simulink model "phase1_PRControl_CIM_noAdapt"  (R2024a)
settings: Solver=VariableStepAuto  StartTime=0.0  StopTime=3  FixedStep=1e-7  MaxStep=1e-6  RelTol=1e-6
values from neighbouring files (symbols this model uses):
  Cf = 22e-6    (= 2.2e-05)    [phase1_PRControl_CIM_noAdapt_init.m]
  L1 = 150e-6    (= 0.00015)    [phase1_PRControl_CIM_noAdapt_init.m]
  L2g = L2+Lg    (= 0.00045)    [phase1_PRControl_CIM_noAdapt_init.m]
  R1 = 0.045    [phase1_PRControl_CIM_noAdapt_init.m]
  R2g = R2+Rg    (= 0.135)    [phase1_PRControl_CIM_noAdapt_init.m]
  Rd = 1    [phase1_PRControl_CIM_noAdapt_init.m]
  w = 2*pi*freq    (= 314.159265359)    [phase1_PRControl_CIM_noAdapt_init.m]
  w2 = 3*w    (= 942.477796077)    [phase1_PRControl_CIM_noAdapt_init.m]
libraries: spsVoltageMeasurementLib x4, spsSeriesRLCBranchLib x3, spsDCVoltageSourceLib x2, cstblocks x2, spsControlledVoltageSourceLib x1, spsCurrentMeasurementLib x1, spsBreakerLib x1, spsPLLLib x1, simulink x1, spsdq0toAlphaBetaZeroLib x1, spsUniversalBridgeLib x1, spspowerguiLib x1
settings Model: Creator=aleks  LastModifiedBy=aleks
settings DataIOCC: ReturnWorkspaceOutputs=off
settings SimscapeCC: SimscapeLogType=all  SimscapeLogOpenViewer=on  SimscapeLogLimitData=off

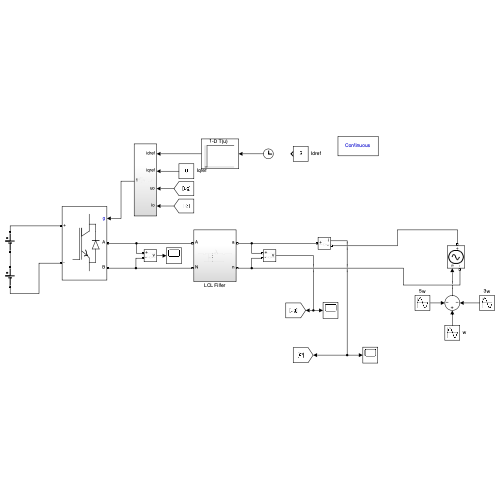
[thumbnail: Simulink's stored preview of the top-level diagram]
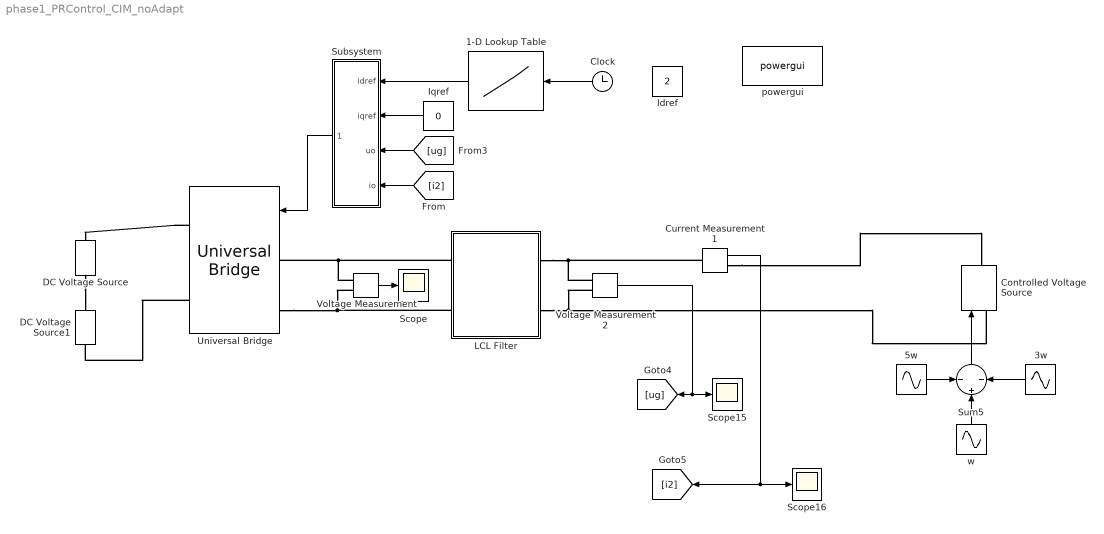
== system phase1_PRControl_CIM_noAdapt ==
  1-D Lookup Table : Lookup_n-D  NumberOfTableDimensions=1  LookupTableObject=''  BreakpointsForDimension1=[0;0.2;0.201;3]  BreakpointsForDimension1FirstPoint=10  BreakpointsForDimension2FirstPoint=10  BreakpointsForDimension1Spacing=12  BreakpointsForDimension2Spacing=12  IndexSearchMethod=Linear search  Table=[0;0;2;2]  DiagnosticForOutOfRangeInput=Error  InternalRulePriority=Speed  RndMeth=Simplest
  3w : Sin  Amplitude=1.5  Frequency=w2  SampleTime=0
  5w : Sin  Amplitude=1.5  Frequency=5*w  SampleTime=0
  Clock : Clock
  Controlled Voltage Source : spsControlledVoltageSourceLib/Controlled Voltage Source  Initialize=on  Source_Type=AC  Amplitude=0  Phase=0  Frequency=0  Measurements=None
  Current Measurement1 : spsCurrentMeasurementLib/Current Measurement  PhasorSimulation=off  OutputType=Complex  PSBequivalent=0
  DC Voltage Source : spsDCVoltageSourceLib/DC Voltage Source  Amplitude=20  Measurements=None
  DC Voltage Source1 : spsDCVoltageSourceLib/DC Voltage Source  Amplitude=20  Measurements=None
  Idref : Constant  Value=2
  Iqref : Constant  Value=0
  LCL Filter : Subsystem
  Scope : Scope
  Scope15 : Scope
  Scope16 : Scope
  Subsystem : Subsystem
  Sum5 : Sum  Inputs=-|+|-
  Universal Bridge : spsUniversalBridgeLib/Universal Bridge  Arms=2  SnubberResistance=1e5  SnubberCapacitance=inf  Device=IGBT / Diodes  Ron=1e-3  Lon=0  ForwardVoltages="[  0  0  ]"  ForwardVoltage=0  GTOparameters=[ 10e-6 , 20e-6 ]  IGBTparameters=[ 1e-6 , 2e-6 ]  Measurements=None  Measurements_2=None  converterType=Rectifier
  Voltage Measurement : spsVoltageMeasurementLib/Voltage Measurement  PhasorSimulation=off  OutputType=Complex  PSBequivalent=0
  Voltage Measurement2 : spsVoltageMeasurementLib/Voltage Measurement  PhasorSimulation=off  OutputType=Complex  PSBequivalent=0
  powergui : spspowerguiLib/powergui  Priority=1  SimulationMode=Continuous  SampleTime=10e-6  frequency=60  Iterations=50  frequencyindice=0  Pbase=100e6  ErrMax=1e-4  UnitsV=kV  UnitsW=MW  buscounter=0  FunctionMessages=off  echomessages=off  EnableUseOfTLC=off  CurrentSourceSwitches=off  DisableSnubberDevices=off  DisableRonSwitches=off  DisableVfSwitches=off  DisplayEquations=off  AutomaticDiscreteSolvers=off  SolverType=Tustin/Backward Euler (TBE)  Interpol=off  ExternalGateDelay=off  methode=off  Ts=100  x0status=blocks  SPID=on  SwTol=0  HookPort=off  NonlinearTolerance=1e-4  nMaxIteration=100  ContinueOnMaxIteration=off  RestoreLinks=warning  ResistiveCurrentMeasurement=off  Frange=[0:2:500]  Ylog=off  Xlog=on  ShowGrid=off  save=off  variable=ZData  structure=0  ZoomFFT=off  StartTime=0.0  cycles=1  DisplayStyle=1  fundamental=60  FreqAxis=off  MaxFrequency=1000  frequencyindicesteady=1  RmsSteady=1  display=off
  w : Sin  Amplitude=15  Frequency=w  SampleTime=0
  wires:
  Voltage Measurement/1 -> Scope/1
  Subsystem/1(1) -> Universal Bridge/1
  [i2] -> Subsystem/4(io)
  [ug] -> Subsystem/3(uo)
  Voltage Measurement2/1 -> [ug], Scope15/1
  Current Measurement1/1 -> Scope16/1, [i2]
  w/1 -> Sum5/2
  3w/1 -> Sum5/3
  5w/1 -> Sum5/1
  Sum5/1 -> Controlled Voltage Source/1
  Iqref/1 -> Subsystem/2(iqref)
  1-D Lookup Table/1 -> Subsystem/1(idref)
  Clock/1 -> 1-D Lookup Table/1
  connections:
  Universal Bridge/RConn1 -- DC Voltage Source/RConn1
  Universal Bridge/RConn2 -- DC Voltage Source1/LConn1
  Voltage Measurement/LConn1 -- LCL Filter/LConn1 -- Universal Bridge/LConn1
  Voltage Measurement2/LConn2 -- Controlled Voltage Source/LConn1 -- LCL Filter/RConn2
  DC Voltage Source/LConn1 -- DC Voltage Source1/RConn1
  Voltage Measurement2/LConn1 -- LCL Filter/RConn1 -- Current Measurement1/LConn1
  Voltage Measurement/LConn2 -- LCL Filter/LConn2 -- Universal Bridge/LConn2
  Current Measurement1/RConn1 -- Controlled Voltage Source/RConn1

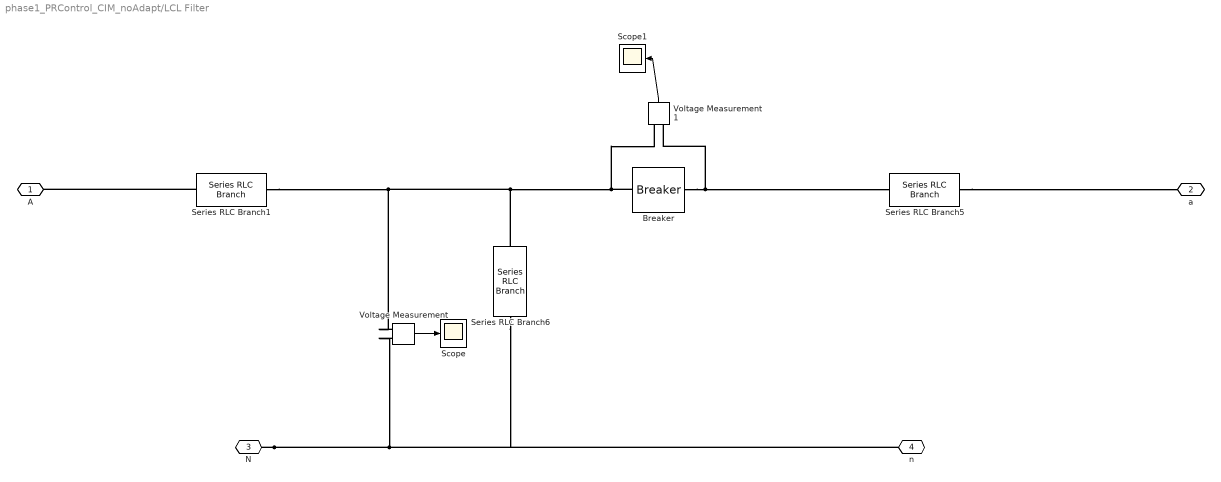
== system phase1_PRControl_CIM_noAdapt/LCL Filter ==
  Breaker : spsBreakerLib/Breaker  InitialState=0  SwitchingTimes=[0.1]  External=off  BreakerResistance=0.0001  SnubberResistance=1e8  SnubberCapacitance=inf  Measurements=None  MoreParameters=on  NoBreakLoop=off
  Scope : Scope
  Scope1 : Scope
  Series RLC Branch1 : spsSeriesRLCBranchLib/Series RLC Branch  LConnTagsString=__new0  RConnTagsString=__new0  BranchType=RL  Resistance=R1  Inductance=L1  SetiL0=off  InitialCurrent=0  Capacitance=1e-6  Setx0=off  InitialVoltage=0  Measurements=None
  Series RLC Branch5 : spsSeriesRLCBranchLib/Series RLC Branch  LConnTagsString=__new0  RConnTagsString=__new0  BranchType=RL  Resistance=R2g  Inductance=L2g  SetiL0=off  InitialCurrent=0  Capacitance=1e-6  Setx0=off  InitialVoltage=0  Measurements=None
  Series RLC Branch6 : spsSeriesRLCBranchLib/Series RLC Branch  LConnTagsString=__new0  RConnTagsString=__new0  BranchType=RC  Resistance=Rd  Inductance=500e-6  SetiL0=off  InitialCurrent=0  Capacitance=Cf  Setx0=off  InitialVoltage=0  Measurements=None
  Voltage Measurement : spsVoltageMeasurementLib/Voltage Measurement  PhasorSimulation=off  OutputType=Complex  PSBequivalent=0
  Voltage Measurement1 : spsVoltageMeasurementLib/Voltage Measurement  PhasorSimulation=off  OutputType=Complex  PSBequivalent=0
  A : PMIOPort  Side=Left
  a : PMIOPort  Port=2  Side=Right
  N : PMIOPort  Port=3  Side=Left
  n : PMIOPort  Port=4  Side=Right
  wires:
  Voltage Measurement1/1 -> Scope1/1
  Voltage Measurement/1 -> Scope/1
  connections:
  N/RConn1 -- Series RLC Branch6/LConn1 -- n/RConn1 -- Voltage Measurement/LConn2
  Series RLC Branch5/RConn1 -- a/RConn1
  Series RLC Branch1/LConn1 -- A/RConn1
  Series RLC Branch6/RConn1 -- Voltage Measurement1/LConn2 -- Breaker/LConn1 -- Voltage Measurement/LConn1 -- Series RLC Branch1/RConn1
  Breaker/RConn1 -- Series RLC Branch5/LConn1 -- Voltage Measurement1/LConn1

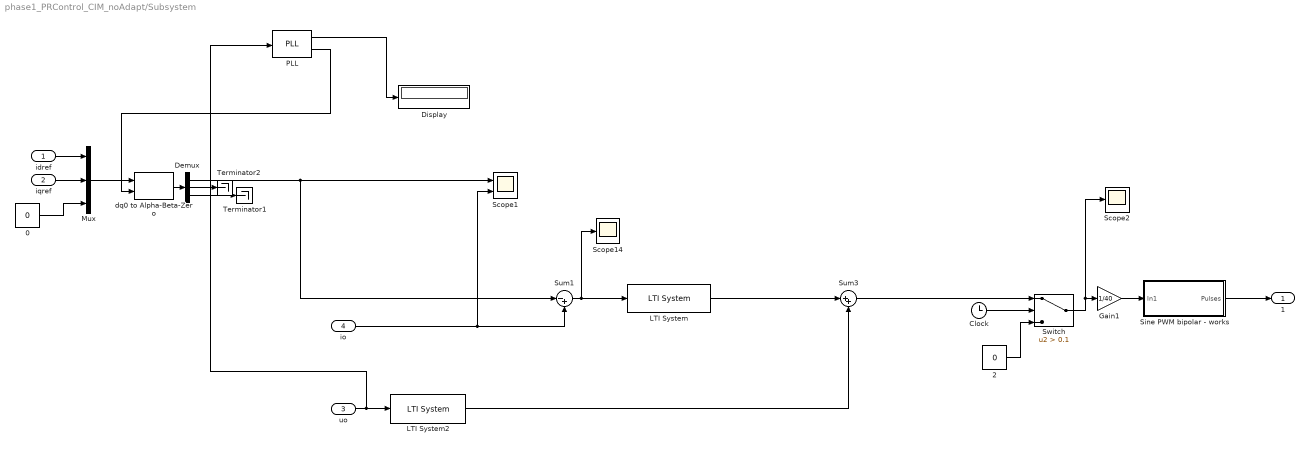
== system phase1_PRControl_CIM_noAdapt/Subsystem ==
  idref : Inport
  iqref : Inport  Port=2
  uo : Inport  Port=3
  io : Inport  Port=4
  0 : Constant  Value=0
  2 : Constant  Value=0
  Clock : Clock
  Demux : Demux  Outputs=3
  Display : Display
  Gain1 : Gain  Gain=1/40
  LTI System : cstblocks/LTI System  sys=R  IC=[]  PadeOrder=0
  LTI System2 : cstblocks/LTI System  sys=Gfffilter  IC=[]  PadeOrder=0
  Mux : Mux  Inputs=3
  PLL : spsPLLLib/PLL  Fmin=49  Par_Init=[0, 50]  ParK=[180, 3200, 1]  TcD=1e-4  MaxRateChangeFreq=12  FilterCutOffFreq=25  Ts=0  AGC=on
      settings: LibrarySourceBlock=sps_lib/Control/PLL
  Scope1 : Scope  NumInputPorts=2
  Scope14 : Scope
  Scope2 : Scope
  Sine PWM bipolar - works : Subsystem
  Sum1 : Sum  Inputs=|-+
  Sum3 : Sum  Inputs=|++
  Switch : Switch  Criteria=u2 > Threshold  Threshold=0.1  SaturateOnIntegerOverflow=off  InputSameDT=off
  Terminator1 : Terminator
  Terminator2 : Terminator
  dq0 to Alpha-Beta-Zero : spsdq0toAlphaBetaZeroLib/dq0 to Alpha-Beta-Zero  Alignment=90 degrees behind phase A axis
  1 : Outport
  wires:
  Demux/1 -> Sum1/1, Scope1/1
  io/1 -> Scope1/2, Sum1/2
  Sine PWM bipolar - works/1(Pulses) -> 1/1
  Gain1/1 -> Sine PWM bipolar - works/1(In1)
  Sum1/1 -> LTI System/1, Scope14/1
  LTI System2/1 -> Sum3/2
  LTI System/1 -> Sum3/1
  uo/1 -> PLL/1, LTI System2/1
  Mux/1 -> dq0 to Alpha-Beta-Zero/1
  0/1 -> Mux/3
  Demux/3 -> Terminator1/1
  Demux/2 -> Terminator2/1
  PLL/1 -> Display/1
  dq0 to Alpha-Beta-Zero/1 -> Demux/1
  PLL/2 -> dq0 to Alpha-Beta-Zero/2
  idref/1 -> Mux/1
  iqref/1 -> Mux/2
  2/1 -> Switch/3
  Clock/1 -> Switch/2
  Switch/1 -> Scope2/1, Gain1/1
  Sum3/1 -> Switch/1

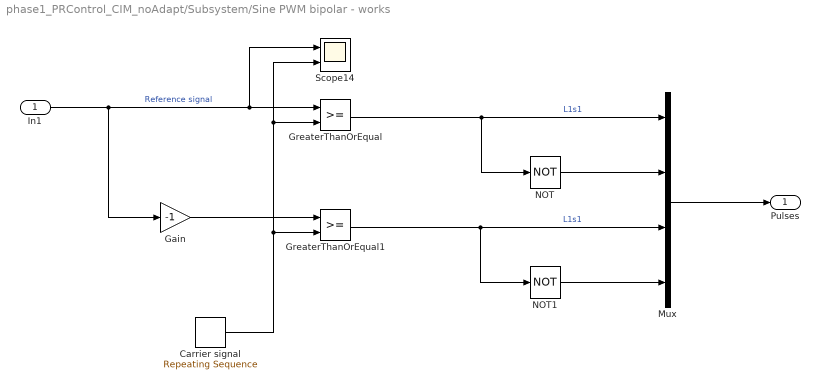
== system phase1_PRControl_CIM_noAdapt/Subsystem/Sine PWM bipolar - works ==
  In1 : Inport
  Carrier signal : simulink/Sources/Repeating Sequence  rep_seq_t=[0 1/24000 1/12000]  rep_seq_y=[-1 1 -1]
  Gain : Gain  Gain=-1
  GreaterThanOrEqual : RelationalOperator  OutDataTypeStr=boolean  RndMeth=Simplest  InputSameDT=off
  GreaterThanOrEqual1 : RelationalOperator  OutDataTypeStr=boolean  RndMeth=Simplest  InputSameDT=off
  Mux : Mux
  NOT : Logic  Operator=NOT  IconShape=distinctive  AllPortsSameDT=off  OutDataTypeStr=boolean
  NOT1 : Logic  Operator=NOT  IconShape=distinctive  AllPortsSameDT=off  OutDataTypeStr=boolean
  Scope14 : Scope  NumInputPorts=2
  Pulses : Outport
  wires:
  Mux/1 -> Pulses/1
  In1/1 -> Scope14/1, GreaterThanOrEqual/1, Gain/1  "Reference signal"
  Carrier signal/1 -> Scope14/2, GreaterThanOrEqual/2, GreaterThanOrEqual1/2
  GreaterThanOrEqual/1 -> NOT/1, Mux/1  "L1s1"
  Gain/1 -> GreaterThanOrEqual1/1
  NOT/1 -> Mux/2
  GreaterThanOrEqual1/1 -> NOT1/1, Mux/3  "L1s1"
  NOT1/1 -> Mux/4
